simulink model "six_plus_six_AcmsteeringV09_main_2lflm"  (R2014a)
settings: Solver=FixedStepDiscrete  StartTime=0.0  StopTime=10.0  FixedStep=0.0005  RelTol=1e-3
InitFcn:
  | Veh_Par_wxt
undefined symbols (not defined in the file or in its folder): acc_spdctl, ag_thr, B, bra_em, bra_pre_gz2, bra_pre_gz34, bra_pre_yd, brakepre_dem_data, brakeTrq_dem_data, bratrq_max, ecucoder_acal, eff_tran, ESP_switch, G, guzhang_lf, guzhang_lm, guzhang_lr, guzhang_rf, guzhang_rm, guzhang_rr, kd1, kd2, ki1, ki2, kp1, kp2, L, myFIS, premax, Radius, RC_switch, s_opt_yi, s_opt_zhuan, s_opt_zhuan_add, s_opt_zhuan_table, spd_map_mot, spd_spdctl, speed_thr_park, TCS_switch, tras_ratio, trq_map_mot, trqmax_yd, trqmax_zx, trqmaxneg, v_gain, v_table, v_thr_park, zhidong_bianmazhi, zhidong_down, zhidong_up, zhidong_youmen, zhuanxiang_bianmazhi, zhuanxiang_down, zhuanxiang_up, zhuanxiang_youmen
libraries: simulink x980, ec5744lib x59, fuzblock x2
(part 23 of 25)

== system six_plus_six_AcmsteeringV09_main_2lflm/MainControl/mode_control/backward/backward/Drive/驱动防滑控制TCS/直行TCS/Subsystem6 ==
  speed_act_lf : Inport
  speed_act_lm : Inport  Port=2
  speed_act_lr : Inport  Port=3
  Gain : Gain  Gain=1/tras_ratio
  Gain1 : Gain  Gain=pi/30
  Gain2 : Gain  Gain=Radius
  Gain3 : Gain  Gain=3.6
  Gain4 : Gain  Gain=v_gain
  MinMax : MinMax  Inputs=3
  v_act_l : Outport
  wires:
  speed_act_lm/1 -> MinMax/2
  speed_act_lr/1 -> MinMax/3
  speed_act_lf/1 -> MinMax/1
  MinMax/1 -> Gain/1
  Gain/1 -> Gain1/1
  Gain1/1 -> Gain2/1
  Gain2/1 -> Gain3/1
  Gain3/1 -> Gain4/1
  Gain4/1 -> v_act_l/1

== system six_plus_six_AcmsteeringV09_main_2lflm/MainControl/mode_control/backward/backward/Drive/驱动防滑控制TCS/直行TCS/Subsystem7 ==
  speed_act_rf : Inport
  speed_act_rm : Inport  Port=2
  speed_act_rr : Inport  Port=3
  Gain : Gain  Gain=1/tras_ratio
  Gain1 : Gain  Gain=pi/30
  Gain2 : Gain  Gain=Radius
  Gain3 : Gain  Gain=3.6
  Gain4 : Gain  Gain=v_gain
  MinMax : MinMax  Inputs=3
  v_act_r : Outport
  wires:
  Gain4/1 -> v_act_r/1
  Gain3/1 -> Gain4/1
  Gain2/1 -> Gain3/1
  Gain1/1 -> Gain2/1
  Gain/1 -> Gain1/1
  MinMax/1 -> Gain/1
  speed_act_rf/1 -> MinMax/1
  speed_act_rr/1 -> MinMax/3
  speed_act_rm/1 -> MinMax/2

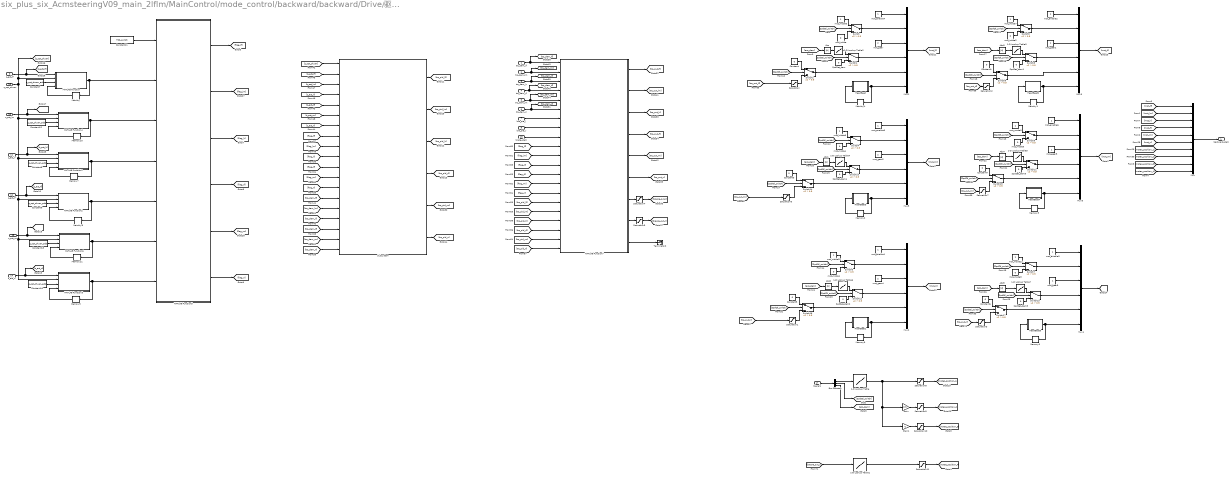
== system six_plus_six_AcmsteeringV09_main_2lflm/MainControl/mode_control/backward/backward/Drive/驱动防滑控制TCS/直行TCS/直行 ==
  trq_dem_lf : Inport
  trq_dem_lm : Inport  Port=2
  trq_dem_lr : Inport  Port=3
  trq_dem_rf : Inport  Port=4
  trq_dem_rm : Inport  Port=5
  trq_dem_rr : Inport  Port=6
  bra_pre_l : Inport  Port=7
  bra_pre_r : Inport  Port=8
  s_act_lf : Inport  Port=9
  s_act_lm : Inport  Port=10
  s_act_lr : Inport  Port=11
  s_act_rf : Inport  Port=12
  s_act_rm : Inport  Port=13
  s_act_rr : Inport  Port=14
  brake_dem : Inport  Port=15
  s_opt_zhuan : Inport  Port=16
  Signals : Inport  Port=17
  1-D Lookup Table : Lookup_n-D  NumberOfTableDimensions=1  BreakpointsForDimension1=zhuanxiang_youmen  Table=zhuanxiang_bianmazhi  InternalRulePriority=Speed  RndMeth=Simplest  InputSameDT=on
  1-D Lookup Table1 : Lookup_n-D  NumberOfTableDimensions=1  BreakpointsForDimension1=zhidong_youmen  Table=zhidong_bianmazhi  InternalRulePriority=Speed  RndMeth=Simplest  InputSameDT=on
  1-D Lookup Table{2..7} (6 alike) : Lookup_n-D  NumberOfTableDimensions=1  BreakpointsForDimension1=acc_spdctl  Table=spd_spdctl  InternalRulePriority=Speed  RndMeth=Simplest  InputSameDT=on
  Abs{,1..5} (6 alike) : Abs
  Bus Selector : BusSelector  OutputSignals=RemoteControl_dem.steer_dem,RemoteControl_dem.SpdCtl_switch,RemoteControl_dem.acc_dem
  Constant{,1,3..6} (6 alike) : Constant  Value=0  OutDataTypeStr=single  SampleTime=-1
  Constant{7..10,12..13} (6 alike) : Constant  Value=s_opt_zhuan_add  OutDataTypeStr=single  SampleTime=-1
  Constant11 : Constant  Value=TCS_switch  OutDataTypeStr=single  SampleTime=-1
  Gain : Gain  Gain=0.5
  Gain1 : Gain  Gain=-1
  HeartBeat : MATLAB Function  TreatAsAtomicUnit=on
  HeartBeat1 : MATLAB Function  TreatAsAtomicUnit=on
  HeartBeat2 : MATLAB Function  TreatAsAtomicUnit=on
  HeartBeat3 : MATLAB Function  TreatAsAtomicUnit=on
  HeartBeat4 : MATLAB Function  TreatAsAtomicUnit=on
  HeartBeat5 : MATLAB Function  TreatAsAtomicUnit=on
  MATLAB Function : MATLAB Function  TreatAsAtomicUnit=on
  MATLAB Function1 : MATLAB Function  TreatAsAtomicUnit=on
  MATLAB Function2 : MATLAB Function  TreatAsAtomicUnit=on
  MATLAB Function3 : MATLAB Function  TreatAsAtomicUnit=on
  MATLAB Function4 : MATLAB Function  TreatAsAtomicUnit=on
  MATLAB Function5 : MATLAB Function  TreatAsAtomicUnit=on
  MATLAB Function6 : MATLAB Function  TreatAsAtomicUnit=on
  MATLAB Function7 : MATLAB Function  TreatAsAtomicUnit=on
  Memory{,1..11} (12 alike) : Memory  InheritSampleTime=on
  Mux : Mux  Inputs=10
  Mux{1..6} (6 alike) : Mux  Inputs=6
  Saturation{,1..3,6..7} (6 alike) : Saturate  UpperLimit=trqmax_zx  LowerLimit=trqmaxneg  OutDataTypeStr=single
  Saturation10 : Saturate  UpperLimit=zhuanxiang_up  LowerLimit=zhuanxiang_down
  Saturation11 : Saturate  UpperLimit=zhidong_up  LowerLimit=zhidong_down
  Saturation4 : Saturate  UpperLimit=premax  LowerLimit=0
  Saturation5 : Saturate  UpperLimit=premax  LowerLimit=0
  Saturation8 : Saturate  UpperLimit=zhuanxiang_up  LowerLimit=zhuanxiang_down
  Saturation9 : Saturate  UpperLimit=zhuanxiang_up  LowerLimit=zhuanxiang_down
  SpdSet_dem{,1..5} (6 alike) : Constant  Value=0  OutDataTypeStr=single  SampleTime=-1
  Subsystem : Subsystem
  Switch{,1..17} (18 alike) : Switch  Criteria=u2 > Threshold  Threshold=0.5
  Terminator2 : Terminator
  mot_enable{1..6} (6 alike) : Constant  OutDataTypeStr=single  SampleTime=-1
  mot_gear : Constant  Value=2  OutDataTypeStr=single  SampleTime=-1
  mot_gear1 : Constant  OutDataTypeStr=single  SampleTime=-1
  mot_gear2 : Constant  Value=2  OutDataTypeStr=single  SampleTime=-1
  mot_gear3 : Constant  OutDataTypeStr=single  SampleTime=-1
  mot_gear4 : Constant  Value=2  OutDataTypeStr=single  SampleTime=-1
  mot_gear5 : Constant  OutDataTypeStr=single  SampleTime=-1
  mot_mode{,1..5} (6 alike) : Constant  Value=0  OutDataTypeStr=single  SampleTime=-1
  mot_mode{6..11} (6 alike) : Constant  OutDataTypeStr=single  SampleTime=-1
  backward_dem : Outport
  wires:
  Mux/1 -> backward_dem/1
  Memory4/1 -> HeartBeat/1(life_pre)
  HeartBeat/1(life) -> Memory4/1, Mux1/6
  Mux1/1 -> [mot_lf]
  [trq_out_lf] -> Saturation/1
  mot_gear/1 -> Mux1/3
  mot_enable4/1 -> Mux1/1
  Switch1/1 -> Mux1/4
  Memory1/1 -> HeartBeat2/1(life_pre)
  HeartBeat2/1(life) -> Mux3/6, Memory1/1
  Mux3/1 -> [mot_rf]
  [trq_out_rf] -> Saturation2/1
  Switch3/1 -> Mux3/2
  mot_gear1/1 -> Mux3/3
  mot_enable2/1 -> Mux3/1
  Switch8/1 -> Mux3/4
  Memory2/1 -> HeartBeat3/1(life_pre)
  HeartBeat3/1(life) -> Mux5/6, Memory2/1
  Mux5/1 -> [mot_lm]
  [trq_out_lm] -> Saturation6/1
  Switch4/1 -> Mux5/2
  mot_gear2/1 -> Mux5/3
  mot_enable5/1 -> Mux5/1
  Switch10/1 -> Mux5/4
  Memory3/1 -> HeartBeat4/1(life_pre)
  HeartBeat4/1(life) -> Memory3/1, Mux6/6
  Mux6/1 -> [mot_rm]
  [trq_out_rm] -> Saturation7/1
  Switch5/1 -> Mux6/2
  mot_gear3/1 -> Mux6/3
  mot_enable6/1 -> Mux6/1
  Switch11/1 -> Mux6/4
  Memory5/1 -> HeartBeat1/1(life_pre)
  HeartBeat1/1(life) -> Mux2/6, Memory5/1
  Mux2/1 -> [mot_lr]
  [trq_out_lr] -> Saturation1/1
  Switch6/1 -> Mux2/2
  mot_gear4/1 -> Mux2/3
  mot_enable1/1 -> Mux2/1
  Switch12/1 -> Mux2/4
  Memory6/1 -> HeartBeat5/1(life_pre)
  HeartBeat5/1(life) -> Memory6/1, Mux4/6
  Mux4/1 -> [mot_rr]
  [trq_out_rr] -> Saturation3/1
  Switch7/1 -> Mux4/2
  mot_gear5/1 -> Mux4/3
  mot_enable3/1 -> Mux4/1
  Switch13/1 -> Mux4/4
  [mot_lf] -> Mux/1
  [mot_lm] -> Mux/2
  [mot_lr] -> Mux/3
  [mot_rf] -> Mux/4
  [mot_rm] -> Mux/5
  [mot_rr] -> Mux/6
  [motec_position_1] -> Mux/7
  [motec_position_2] -> Mux/8
  [motec_position_3] -> Mux/9
  1-D Lookup Table1/1 -> Saturation11/1
  1-D Lookup Table/1 -> Gain1/1, Gain/1, Saturation8/1
  Signals/1 -> Bus Selector/1
  Gain1/1 -> Saturation10/1
  Bus Selector/1 -> 1-D Lookup Table/1  "<steer_dem>"
  Gain/1 -> Saturation9/1
  Saturation8/1 -> [motec_position_1]
  Saturation9/1 -> [motec_position_2]
  Saturation10/1 -> [motec_position_3]
  Saturation11/1 -> [motec_position_4]
  [brapre_out_l] -> 1-D Lookup Table1/1
  [motec_position_4] -> Mux/10
  Bus Selector/2 -> [SpdCtl_switch]  "<SpdCtl_switch>"
  [SpdCtl_switch] -> Switch/2
  mot_mode6/1 -> Switch/1
  mot_mode/1 -> Switch/3
  Switch/1 -> Mux1/2
  [SpdCtl_switch] -> Switch1/2
  SpdSet_dem/1 -> Switch1/3
  Bus Selector/3 -> [acc_dem]  "<acc_dem>"
  [acc_dem] -> Abs/1
  1-D Lookup Table2/1 -> Switch1/1
  [SpdCtl_switch] -> Switch2/2
  Saturation/1 -> Switch2/3
  Constant/1 -> Switch2/1
  Switch2/1 -> Mux1/5
  [SpdCtl_switch] -> Switch3/2
  mot_mode7/1 -> Switch3/1
  mot_mode2/1 -> Switch3/3
  [SpdCtl_switch] -> Switch4/2
  mot_mode8/1 -> Switch4/1
  mot_mode4/1 -> Switch4/3
  [SpdCtl_switch] -> Switch5/2
  mot_mode9/1 -> Switch5/1
  mot_mode5/1 -> Switch5/3
  [SpdCtl_switch] -> Switch6/2
  mot_mode10/1 -> Switch6/1
  mot_mode1/1 -> Switch6/3
  [SpdCtl_switch] -> Switch7/2
  mot_mode11/1 -> Switch7/1
  mot_mode3/1 -> Switch7/3
  [SpdCtl_switch] -> Switch8/2
  [acc_dem] -> Abs3/1
  1-D Lookup Table3/1 -> Switch8/1
  SpdSet_dem1/1 -> Switch8/3
  [SpdCtl_switch] -> Switch9/2
  Constant1/1 -> Switch9/1
  Saturation2/1 -> Switch9/3
  Switch9/1 -> Mux3/5
  [SpdCtl_switch] -> Switch10/2
  [acc_dem] -> Abs1/1
  1-D Lookup Table4/1 -> Switch10/1
  SpdSet_dem4/1 -> Switch10/3
  [SpdCtl_switch] -> Switch11/2
  [acc_dem] -> Abs4/1
  1-D Lookup Table5/1 -> Switch11/1
  SpdSet_dem5/1 -> Switch11/3
  [SpdCtl_switch] -> Switch12/2
  [acc_dem] -> Abs2/1
  1-D Lookup Table6/1 -> Switch12/1
  SpdSet_dem2/1 -> Switch12/3
  [SpdCtl_switch] -> Switch13/2
  [acc_dem] -> Abs5/1
  1-D Lookup Table7/1 -> Switch13/1
  SpdSet_dem3/1 -> Switch13/3
  [SpdCtl_switch] -> Switch14/2
  Constant3/1 -> Switch14/1
  Saturation6/1 -> Switch14/3
  Switch14/1 -> Mux5/5
  [SpdCtl_switch] -> Switch15/2
  Constant4/1 -> Switch15/1
  Saturation7/1 -> Switch15/3
  Switch15/1 -> Mux6/5
  [SpdCtl_switch] -> Switch16/2
  Constant5/1 -> Switch16/1
  Saturation1/1 -> Switch16/3
  Switch16/1 -> Mux2/5
  [SpdCtl_switch] -> Switch17/2
  Constant6/1 -> Switch17/1
  Saturation3/1 -> Switch17/3
  Switch17/1 -> Mux4/5
  Constant10/1 -> MATLAB Function3/3(s_opt_zhuan_add)
  Memory9/1 -> MATLAB Function3/4(flag_rr_pre)
  MATLAB Function3/1(flag_rr) -> Memory9/1, MATLAB Function5/7(flag_rr)
  s_act_rr/1 -> [s_act_rr], MATLAB Function3/1(s_act_rr)
  Constant9/1 -> MATLAB Function2/3(s_opt_zhuan_add)
  Memory8/1 -> MATLAB Function2/4(flag_rf_pre)
  MATLAB Function2/1(flag_rf) -> Memory8/1, MATLAB Function5/5(flag_rf)
  s_act_rf/1 -> MATLAB Function2/1(s_act_rf), [s_act_rf]
  Constant8/1 -> MATLAB Function1/3(s_opt_zhuan_add)
  Memory7/1 -> MATLAB Function1/4(flag_lr_pre)
  MATLAB Function1/1(flag_lr) -> Memory7/1, MATLAB Function5/4(flag_lr)
  s_act_lr/1 -> [s_act_lr], MATLAB Function1/1(s_act_lr)
  Constant7/1 -> MATLAB Function/3(s_opt_zhuan_add)
  Memory/1 -> MATLAB Function/4(flag_lf_pre)
  MATLAB Function/1(flag_lf) -> Memory/1, MATLAB Function5/2(flag_lf)
  s_act_lf/1 -> [s_act_lf], MATLAB Function/1(s_act_lf)
  [trq_dem_lf] -> Subsystem/14(trq_dem_lf)
  [flag_lf] -> Subsystem/8(flag_lf)
  [trq_dem_rf] -> Subsystem/17(trq_dem_rf)
  [trq_dem_lr] -> Subsystem/16(trq_dem_lr)
  [flag_lr] -> Subsystem/10(flag_lr)
  [flag_rf] -> Subsystem/11(flag_rf)
  [trq_dem_rr] -> Subsystem/19(trq_dem_rr)
  [flag_rr] -> Subsystem/13(flag_rr)
  [s_opt_zhuan] -> Subsystem/1(s_opt_zhuan)
  [s_act_rr] -> Subsystem/7(s_act_rr)
  [s_act_rf] -> Subsystem/5(s_act_rf)
  [s_act_lr] -> Subsystem/4(s_act_lr)
  [s_act_lf] -> Subsystem/2(s_act_lf)
  Subsystem/3(trq_pid_lr) -> [trq_pid_lr]
  Subsystem/1(trq_pid_lf) -> [trq_pid_lf]
  Subsystem/6(trq_pid_rr) -> [trq_pid_rr]
  Subsystem/4(trq_pid_rf) -> [trq_pid_rf]
  MATLAB Function5/1(flag_lf1) -> [flag_lf]
  MATLAB Function5/3(flag_lr1) -> [flag_lr]
  MATLAB Function5/4(flag_rf1) -> [flag_rf]
  MATLAB Function5/6(flag_rr1) -> [flag_rr]
  Constant12/1 -> MATLAB Function4/3(s_opt_zhuan_add)
  Memory10/1 -> MATLAB Function4/4(flag_lm_pre)
  MATLAB Function4/1(flag_lm) -> MATLAB Function5/3(flag_lm), Memory10/1
  s_act_lm/1 -> MATLAB Function4/1(s_act_lm), [s_act_lm]
  Constant13/1 -> MATLAB Function6/3(s_opt_zhuan_add)
  Memory11/1 -> MATLAB Function6/4(flag_rm_pre)
  MATLAB Function6/1(flag_rm) -> Memory11/1, MATLAB Function5/6(flag_rm)
  s_act_rm/1 -> [s_act_rm], MATLAB Function6/1(s_act_rm)
  s_opt_zhuan/1 -> MATLAB Function/2(s_opt_zhuan), [s_opt_zhuan], MATLAB Function4/2(s_opt_zhuan), MATLAB Function1/2(s_opt_zhuan), MATLAB Function2/2(s_opt_zhuan), MATLAB Function6/2(s_opt_zhuan), MATLAB Function3/2(s_opt_zhuan)
  MATLAB Function5/2(flag_lm1) -> [flag_lm]
  MATLAB Function5/5(flag_rm1) -> [flag_rm]
  Constant11/1 -> MATLAB Function5/1(TCS_switch)
  [s_act_lm] -> Subsystem/3(s_act_lm)
  [s_act_rm] -> Subsystem/6(s_act_rm)
  [flag_lm] -> Subsystem/9(flag_lm)
  [flag_rm] -> Subsystem/12(flag_rm)
  [trq_dem_lm] -> Subsystem/15(trq_dem_lm)
  [trq_dem_rm] -> Subsystem/18(trq_dem_rm)
  Subsystem/2(trq_pid_lm) -> [trq_pid_lm]
  Subsystem/5(trq_pid_rm) -> [trq_pid_rm]
  [flag_rr] -> MATLAB Function7/15(flag_rr)
  [flag_rf] -> MATLAB Function7/13(flag_rf)
  [flag_lr] -> MATLAB Function7/12(flag_lr)
  [flag_lf] -> MATLAB Function7/10(flag_lf)
  [trq_pid_lf] -> MATLAB Function7/16(trq_pid_lf)
  [trq_pid_lr] -> MATLAB Function7/18(trq_pid_lr)
  [trq_pid_rf] -> MATLAB Function7/19(trq_pid_rf)
  [trq_pid_rr] -> MATLAB Function7/21(trq_pid_rr)
  trq_dem_lf/1 -> MATLAB Function7/1(trq_dem_lf), [trq_dem_lf]
  trq_dem_lr/1 -> [trq_dem_lr], MATLAB Function7/3(trq_dem_lr)
  trq_dem_rf/1 -> MATLAB Function7/4(trq_dem_rf), [trq_dem_rf]
  trq_dem_rr/1 -> [trq_dem_rr], MATLAB Function7/6(trq_dem_rr)
  bra_pre_l/1 -> MATLAB Function7/7(bra_pre_l)
  bra_pre_r/1 -> MATLAB Function7/8(bra_pre_r)
  MATLAB Function7/1(trq_out_lf) -> [trq_out_lf]
  MATLAB Function7/3(trq_out_lr) -> [trq_out_lr]
  MATLAB Function7/4(trq_out_rf) -> [trq_out_rf]
  MATLAB Function7/6(trq_out_rr) -> [trq_out_rr]
  MATLAB Function7/7(brapre_out_l) -> Saturation4/1
  MATLAB Function7/8(brapre_out_r) -> Saturation5/1
  brake_dem/1 -> MATLAB Function7/9(brake_dem)
  MATLAB Function7/9(mode) -> Terminator2/1
  Saturation4/1 -> [brapre_out_l]
  Saturation5/1 -> [brapre_out_r]
  MATLAB Function7/2(trq_out_lm) -> [trq_out_lm]
  MATLAB Function7/5(trq_out_rm) -> [trq_out_rm]
  trq_dem_lm/1 -> [trq_dem_lm], MATLAB Function7/2(trq_dem_lm)
  trq_dem_rm/1 -> [trq_dem_rm], MATLAB Function7/5(trq_dem_rm)
  [flag_lm] -> MATLAB Function7/11(flag_lm)
  [flag_rm] -> MATLAB Function7/14(flag_rm)
  [trq_pid_lm] -> MATLAB Function7/17(trq_pid_lm)
  [trq_pid_rm] -> MATLAB Function7/20(trq_pid_rm)
  Abs/1 -> 1-D Lookup Table2/1
  Abs1/1 -> 1-D Lookup Table4/1
  Abs2/1 -> 1-D Lookup Table6/1
  Abs3/1 -> 1-D Lookup Table3/1
  Abs4/1 -> 1-D Lookup Table5/1
  Abs5/1 -> 1-D Lookup Table7/1

== system six_plus_six_AcmsteeringV09_main_2lflm/MainControl/mode_control/forward/forward/Drive/驱动防滑控制TCS/直行TCS/Subsystem ==
  speed_act_lf : Inport
  v_act : Inport  Port=2
  Add : Sum
  Constant : Constant  Value=eps  OutDataTypeStr=single  SampleTime=-1
  Divide : Product  Inputs=*/
  Gain : Gain  Gain=pi/30
  Gain1 : Gain  Gain=Radius
  Gain2 : Gain  Gain=1/3.6
  Gain3 : Gain  Gain=1/tras_ratio
  Subtract : Sum  Inputs=+-
  s_act_lf : Outport
  wires:
  Divide/1 -> s_act_lf/1
  Add/1 -> Divide/2
  Constant/1 -> Add/2
  Subtract/1 -> Divide/1
  Gain1/1 -> Subtract/1, Add/1
  v_act/1 -> Gain2/1
  Gain/1 -> Gain1/1
  speed_act_lf/1 -> Gain3/1
  Gain3/1 -> Gain/1
  Gain2/1 -> Subtract/2

== system six_plus_six_AcmsteeringV09_main_2lflm/MainControl/mode_control/forward/forward/Drive/驱动防滑控制TCS/直行TCS/Subsystem1 ==
  speed_act_lm : Inport
  v_act : Inport  Port=2
  Add : Sum
  Constant : Constant  Value=eps  OutDataTypeStr=single  SampleTime=-1
  Divide : Product  Inputs=*/
  Gain : Gain  Gain=pi/30
  Gain1 : Gain  Gain=Radius
  Gain2 : Gain  Gain=1/3.6
  Gain3 : Gain  Gain=1/tras_ratio
  Subtract : Sum  Inputs=+-
  s_act_lm : Outport
  wires:
  Gain2/1 -> Subtract/2
  Gain3/1 -> Gain/1
  speed_act_lm/1 -> Gain3/1
  Gain/1 -> Gain1/1
  v_act/1 -> Gain2/1
  Gain1/1 -> Add/1, Subtract/1
  Subtract/1 -> Divide/1
  Constant/1 -> Add/2
  Add/1 -> Divide/2
  Divide/1 -> s_act_lm/1

== system six_plus_six_AcmsteeringV09_main_2lflm/MainControl/mode_control/forward/forward/Drive/驱动防滑控制TCS/直行TCS/Subsystem2 ==
  speed_act_lr : Inport
  v_act : Inport  Port=2
  Add : Sum
  Constant : Constant  Value=eps  OutDataTypeStr=single  SampleTime=-1
  Divide : Product  Inputs=*/
  Gain : Gain  Gain=pi/30
  Gain1 : Gain  Gain=Radius
  Gain2 : Gain  Gain=1/3.6
  Gain3 : Gain  Gain=1/tras_ratio
  Subtract : Sum  Inputs=+-
  s_act_lr : Outport
  wires:
  Gain2/1 -> Subtract/2
  Gain3/1 -> Gain/1
  speed_act_lr/1 -> Gain3/1
  Gain/1 -> Gain1/1
  v_act/1 -> Gain2/1
  Gain1/1 -> Add/1, Subtract/1
  Subtract/1 -> Divide/1
  Constant/1 -> Add/2
  Add/1 -> Divide/2
  Divide/1 -> s_act_lr/1

== system six_plus_six_AcmsteeringV09_main_2lflm/MainControl/mode_control/forward/forward/Drive/驱动防滑控制TCS/直行TCS/Subsystem3 ==
  speed_act_rf : Inport
  v_act : Inport  Port=2
  Add : Sum
  Constant : Constant  Value=eps  OutDataTypeStr=single  SampleTime=-1
  Divide : Product  Inputs=*/
  Gain : Gain  Gain=pi/30
  Gain1 : Gain  Gain=Radius
  Gain2 : Gain  Gain=1/3.6
  Gain3 : Gain  Gain=1/tras_ratio
  Subtract : Sum  Inputs=+-
  s_act_rf : Outport
  wires:
  Divide/1 -> s_act_rf/1
  Add/1 -> Divide/2
  Constant/1 -> Add/2
  Subtract/1 -> Divide/1
  Gain1/1 -> Subtract/1, Add/1
  v_act/1 -> Gain2/1
  Gain/1 -> Gain1/1
  speed_act_rf/1 -> Gain3/1
  Gain3/1 -> Gain/1
  Gain2/1 -> Subtract/2

== system six_plus_six_AcmsteeringV09_main_2lflm/MainControl/mode_control/forward/forward/Drive/驱动防滑控制TCS/直行TCS/Subsystem4 ==
  speed_act_rm : Inport
  v_act : Inport  Port=2
  Add : Sum
  Constant : Constant  Value=eps  OutDataTypeStr=single  SampleTime=-1
  Divide : Product  Inputs=*/
  Gain : Gain  Gain=pi/30
  Gain1 : Gain  Gain=Radius
  Gain2 : Gain  Gain=1/3.6
  Gain3 : Gain  Gain=1/tras_ratio
  Subtract : Sum  Inputs=+-
  s_act_rm : Outport
  wires:
  Gain2/1 -> Subtract/2
  Gain3/1 -> Gain/1
  speed_act_rm/1 -> Gain3/1
  Gain/1 -> Gain1/1
  v_act/1 -> Gain2/1
  Gain1/1 -> Add/1, Subtract/1
  Subtract/1 -> Divide/1
  Constant/1 -> Add/2
  Add/1 -> Divide/2
  Divide/1 -> s_act_rm/1

== system six_plus_six_AcmsteeringV09_main_2lflm/MainControl/mode_control/forward/forward/Drive/驱动防滑控制TCS/直行TCS/Subsystem5 ==
  speed_act_rr : Inport
  v_act : Inport  Port=2
  Add : Sum
  Constant : Constant  Value=eps  OutDataTypeStr=single  SampleTime=-1
  Divide : Product  Inputs=*/
  Gain : Gain  Gain=pi/30
  Gain1 : Gain  Gain=Radius
  Gain2 : Gain  Gain=1/3.6
  Gain3 : Gain  Gain=1/tras_ratio
  Subtract : Sum  Inputs=+-
  s_act_rr : Outport
  wires:
  Divide/1 -> s_act_rr/1
  Add/1 -> Divide/2
  Constant/1 -> Add/2
  Subtract/1 -> Divide/1
  Gain1/1 -> Subtract/1, Add/1
  v_act/1 -> Gain2/1
  Gain/1 -> Gain1/1
  speed_act_rr/1 -> Gain3/1
  Gain3/1 -> Gain/1
  Gain2/1 -> Subtract/2

== system six_plus_six_AcmsteeringV09_main_2lflm/MainControl/mode_control/forward/forward/Drive/驱动防滑控制TCS/直行TCS/Subsystem6 ==
  speed_act_lf : Inport
  speed_act_lm : Inport  Port=2
  speed_act_lr : Inport  Port=3
  Gain : Gain  Gain=1/tras_ratio
  Gain1 : Gain  Gain=pi/30
  Gain2 : Gain  Gain=Radius
  Gain3 : Gain  Gain=3.6
  Gain4 : Gain  Gain=v_gain
  MinMax : MinMax  Inputs=3
  v_act_l : Outport
  wires:
  speed_act_lm/1 -> MinMax/2
  speed_act_lr/1 -> MinMax/3
  speed_act_lf/1 -> MinMax/1
  MinMax/1 -> Gain/1
  Gain/1 -> Gain1/1
  Gain1/1 -> Gain2/1
  Gain2/1 -> Gain3/1
  Gain3/1 -> Gain4/1
  Gain4/1 -> v_act_l/1

== system six_plus_six_AcmsteeringV09_main_2lflm/MainControl/mode_control/forward/forward/Drive/驱动防滑控制TCS/直行TCS/Subsystem7 ==
  speed_act_rf : Inport
  speed_act_rm : Inport  Port=2
  speed_act_rr : Inport  Port=3
  Gain : Gain  Gain=1/tras_ratio
  Gain1 : Gain  Gain=pi/30
  Gain2 : Gain  Gain=Radius
  Gain3 : Gain  Gain=3.6
  Gain4 : Gain  Gain=v_gain
  MinMax : MinMax  Inputs=3
  v_act_r : Outport
  wires:
  Gain4/1 -> v_act_r/1
  Gain3/1 -> Gain4/1
  Gain2/1 -> Gain3/1
  Gain1/1 -> Gain2/1
  Gain/1 -> Gain1/1
  MinMax/1 -> Gain/1
  speed_act_rf/1 -> MinMax/1
  speed_act_rr/1 -> MinMax/3
  speed_act_rm/1 -> MinMax/2

== matlab function six_plus_six_AcmsteeringV09_main_2lflm/MainControl/mode_control/neutral/neutral/HeartBeat ==
  data: life_pre input; life output
function life = fcn(life_pre)
%#codegen
life=single(life_pre+1);
if life>255
    life=single(0);
end
end

== matlab function six_plus_six_AcmsteeringV09_main_2lflm/MainControl/mode_control/neutral/neutral/HeartBeat1 ==
  data: life_pre input; life output
function life = fcn(life_pre)
%#codegen
life=single(life_pre+1);
if life>255
    life=single(0);
end
end

== matlab function six_plus_six_AcmsteeringV09_main_2lflm/MainControl/mode_control/neutral/neutral/HeartBeat2 ==
  data: life_pre input; life output
function life = fcn(life_pre)
%#codegen
life=single(life_pre+1);
if life>255
    life=single(0);
end
end

== matlab function six_plus_six_AcmsteeringV09_main_2lflm/MainControl/mode_control/backward/backward/Brake/HeartBeat ==
  data: life_pre input; life output
function life = fcn(life_pre)
%#codegen
life=single(life_pre+1);
if life>255
    life=single(0);
end
end

== matlab function six_plus_six_AcmsteeringV09_main_2lflm/MainControl/mode_control/backward/backward/Brake/HeartBeat2 ==
  data: life_pre input; life output
function life = fcn(life_pre)
%#codegen
life=single(life_pre+1);
if life>255
    life=single(0);
end
end

== matlab function six_plus_six_AcmsteeringV09_main_2lflm/MainControl/mode_control/backward/backward/Brake/HeartBeat4 ==
  data: life_pre input; life output
function life = fcn(life_pre)
%#codegen
life=single(life_pre+1);
if life>255
    life=single(0);
end
end

== matlab function six_plus_six_AcmsteeringV09_main_2lflm/MainControl/mode_control/backward/backward/Brake/Switch Case Action Subsystem/MATLAB Function5 ==
  data: bratrq_dem_lf input; bratrq_dem_lm input; bratrq_dem_lr input; bratrq_dem_rf input; bratrq_dem_rm input; bratrq_dem_rr input; pwr_chg_bat input; bratrq_mot_lf output; bratrq_mot_lm output; pwr_chg_bat1 input; pwr_chg_bat2 input; trqlimL_dig_lf input; bratrq_mot_lr output; bratrq_mot_rf output; bratrq_mot_rm output; bratrq_mot_rr output; trqlimL_dig_lm input; trqlimL_dig_lr input; trqlimL_dig_rf input; trqlimL_dig_rm input; trqlimL_dig_rr input; speed_act_lf input; speed_act_lm input; speed_act_lr input; speed_act_rf input; speed_act_rm input; speed_act_rr input; trqlim_map_lf input; brapre_out_l output; brapre_out_r output; trqlim_map_lm input; trqlim_map_lr input; trqlim_map_rf input; trqlim_map_rm input; trqlim_map_rr input; tras_ratio input; guzhang_lf input; guzhang_lm input; guzhang_lr input; guzhang_rf input; guzhang_rm input; guzhang_rr input
function [bratrq_mot_lf,bratrq_mot_lm,bratrq_mot_lr,bratrq_mot_rf,bratrq_mot_rm,bratrq_mot_rr,brapre_out_l,brapre_out_r] = fcn(bratrq_dem_lf,bratrq_dem_lm,bratrq_dem_lr,bratrq_dem_rf,bratrq_dem_rm,bratrq_dem_rr,pwr_chg_bat,pwr_chg_bat1,pwr_chg_bat2,trqlimL_dig_lf,trqlimL_dig_lm,trqlimL_dig_lr,trqlimL_dig_rf,trqlimL_dig_rm,trqlimL_dig_rr,speed_act_lf,speed_act_lm,speed_act_lr,speed_act_rf,speed_act_rm,speed_act_rr,trqlim_map_lf,trqlim_map_lm,trqlim_map_lr,trqlim_map_rf,trqlim_map_rm,trqlim_map_rr,tras_ratio,guzhang_lf,guzhang_lm,guzhang_lr,guzhang_rf,guzhang_rm,guzhang_rr)
%#codegen pid模块在外面做，里面进行十六种情况的判断，先看一下效果，不能再修改。前轴单独控制，后轴低选控制

bratrq_mot_lf1=single(bratrq_dem_lf/tras_ratio);
bratrq_mot_lf2=single(9549*(pwr_chg_bat/2)/speed_act_lf);
bratrq_mot_lf=single(min(trqlimL_dig_lf,min(bratrq_mot_lf1,bratrq_mot_lf2)));

bratrq_mot_lm1=single(bratrq_dem_lm/tras_ratio);
bratrq_mot_lm2=single(9549*(pwr_chg_bat1/2)/speed_act_lm);
bratrq_mot_lm=single(min(trqlimL_dig_lm,min(bratrq_mot_lm1,bratrq_mot_lm2)));

bratrq_mot_lr1=single(bratrq_dem_lr/tras_ratio);
bratrq_mot_lr2=single(9549*(pwr_chg_bat2/2)/speed_act_lr);
bratrq_mot_lr=single(min(trqlimL_dig_lr,min(bratrq_mot_lr1,bratrq_mot_lr2)));
 
bratrq_mot_rf1=single(bratrq_dem_rf/tras_ratio);
bratrq_mot_rf2=single(9549*(pwr_chg_bat/2)/speed_act_rf);
bratrq_mot_rf=single(min(trqlimL_dig_rf,min(bratrq_mot_rf1,bratrq_mot_rf2)));

bratrq_mot_rm1=single(bratrq_dem_rm/tras_ratio);
bratrq_mot_rm2=single(9549*(pwr_chg_bat1/2)/speed_act_rm);
bratrq_mot_rm=single(min(trqlimL_dig_rm,min(bratrq_mot_rm1,bratrq_mot_rm2)));

bratrq_mot_rr1=single(bratrq_dem_rr/tras_ratio);
bratrq_mot_rr2=single(9549*(pwr_chg_bat2/2)/speed_act_rr);
bratrq_mot_rr=single(min(trqlimL_dig_rr,min(bratrq_mot_rr1,bratrq_mot_rr2)));

brapre_out_l=single(((bratrq_dem_lf+bratrq_dem_lm+bratrq_dem_lr)-(bratrq_mot_lf+bratrq_mot_lm+bratrq_mot_lr)*tras_ratio)/3/150);
brapre_out_r=single(((bratrq_dem_rf+bratrq_dem_rm+bratrq_dem_rr)-(bratrq_mot_rf+bratrq_mot_rm+bratrq_mot_rr)*tras_ratio)/3/150);







bratrq_mot_lf=single(min(bratrq_mot_lf,trqlim_map_lf));%限一下最大值在外特性内，最小值大于0
bratrq_mot_lf=single(max(bratrq_mot_lf,0));
bratrq_mot_lr=single(min(bratrq_mot_lr,trqlim_map_lr));
bratrq_mot_lr=single(max(bratrq_mot_lr,0));
bratrq_mot_rf=single(min(bratrq_mot_rf,trqlim_map_rf));
bratrq_mot_rf=single(max(bratrq_mot_rf,0));
bratrq_mot_rr=single(min(bratrq_mot_rr,trqlim_map_rr));
bratrq_mot_rr=single(max(bratrq_mot_rr,0));

% brapre_out_l=brapre_out_l;
% brapre_out_r=brapre_out_r;
brapre_out_l=single(brapre_out_l*150/125);%第二辆车的制动压力与制动力的关系调整一下。
brapre_out_r=single(brapre_out_r*150/125);

if guzhang_lf==1
    bratrq_mot_lf=single(0);
end
if guzhang_lm==1
    bratrq_mot_lm=single(0);
end
if guzhang_lr==1
    bratrq_mot_lr=single(0);
end
if guzhang_rf==1
    bratrq_mot_rf=single(0);
end
if guzhang_rm==1
    bratrq_mot_rm=single(0);
end
if guzhang_rr==1
    bratrq_mot_rr=single(0);
end

end

== matlab function six_plus_six_AcmsteeringV09_main_2lflm/MainControl/mode_control/center_steer/center_steer/HeartBeat4 ==
  data: life_pre input; life output
function life = fcn(life_pre)
%#codegen
life=single(life_pre+1);
if life>255
    life=single(0);
end
end

== matlab function six_plus_six_AcmsteeringV09_main_2lflm/MainControl/mode_control/emergency_stop/emergency_stop/HeartBeat2 ==
  data: life_pre input; life output
function life = fcn(life_pre)
%#codegen
life=single(life_pre+1);
if life>255
    life=single(0);
end
end

== matlab function six_plus_six_AcmsteeringV09_main_2lflm/MainControl/mode_control/forward/forward/Drive/驱动防滑控制TCS/直行TCS/直行/HeartBeat ==
  data: life_pre input; life output
function life = fcn(life_pre)
%#codegen
life=single(life_pre+1);
if life>255
    life=single(0);
end
end

== matlab function six_plus_six_AcmsteeringV09_main_2lflm/MainControl/mode_switch/mode_switch ==
  data: brake_emerg input; park input; mode_dem_out output int8; acc_dem input; steer_dem input; brake_dem input; center input; MCU0_SpeedFdk input; MCU0_1SpeedFdk input; MCU0_2SpeedFdk input; MCU0_3SpeedFdk input; MCU0_4SpeedFdk input; MCU0_5SpeedFdk input; speed_thr_park input; mode_dem_out_pre input
 function mode_dem_out = fcn(brake_emerg,park,acc_dem,steer_dem,brake_dem,center,MCU0_SpeedFdk,MCU0_1SpeedFdk,MCU0_2SpeedFdk,MCU0_3SpeedFdk,MCU0_4SpeedFdk,MCU0_5SpeedFdk,speed_thr_park,mode_dem_out_pre)
%#codegen
mode_dem_out=int8(mode_dem_out_pre);

if park==1  && MCU0_SpeedFdk<=speed_thr_park && MCU0_1SpeedFdk<=speed_thr_park && MCU0_2SpeedFdk<=speed_thr_park && MCU0_3SpeedFdk<=speed_thr_park  && MCU0_4SpeedFdk<=speed_thr_park  && MCU0_5SpeedFdk<=speed_thr_park && brake_emerg==0
    mode_dem_out=int8(0);
elseif acc_dem>0 && MCU0_SpeedFdk>=0 && MCU0_1SpeedFdk>=0 && MCU0_2SpeedFdk>=0 && MCU0_3SpeedFdk>=0  && MCU0_4SpeedFdk>=0  && MCU0_5SpeedFdk>=0 && brake_emerg==0  && park==0  && center==0
    mode_dem_out=int8(1);
elseif acc_dem==0 && brake_emerg==0  && park==0  && center==0
    mode_dem_out=int8(2);
elseif acc_dem<0 && MCU0_SpeedFdk>=0 && MCU0_1SpeedFdk>=0 && MCU0_2SpeedFdk>=0 && MCU0_3SpeedFdk>=0  && MCU0_4SpeedFdk>=0  && MCU0_5SpeedFdk>=0 && brake_emerg==0  && park==0  && center==0
    mode_dem_out=int8(3);
elseif center==1  && brake_emerg==0  && park==0        
    mode_dem_out=int8(1);
elseif brake_emerg==1
    mode_dem_out=int8(5);   
% else
%     mode_dem_out=int8(5);
end



end

== matlab function six_plus_six_AcmsteeringV09_main_2lflm/Data_input/6/Enabled
Subsystem/MATLAB Function ==
  data: data1 input; y output; data2 input; data3 input; data4 input
function y = fcn(data1,data2,data3,data4)
%#codegen
y1=data4*256^3+data3*256^2+data2*256+data1;
y=typecast(uint32(y1),'single');
end
% y = u;

== matlab function six_plus_six_AcmsteeringV09_main_2lflm/Data_input/9/Enabled Subsystem/MATLAB Function1 ==
  data: data1 input; y output; data2 input; data3 input; data4 input
function y = fcn(data1,data2,data3,data4)
%#codegen
y1=data4*256^3+data3*256^2+data2*256+data1;
% y=typecast(uint32(y1),'single');
y=single(y1*10^-7);
end
% y = u;

== matlab function six_plus_six_AcmsteeringV09_main_2lflm/MainControl/mode_control/Park/park/HeartBeat2 ==
  data: life_pre input; life output
function life = fcn(life_pre)
%#codegen
life=single(life_pre+1);
if life>255
    life=single(0);
end
end

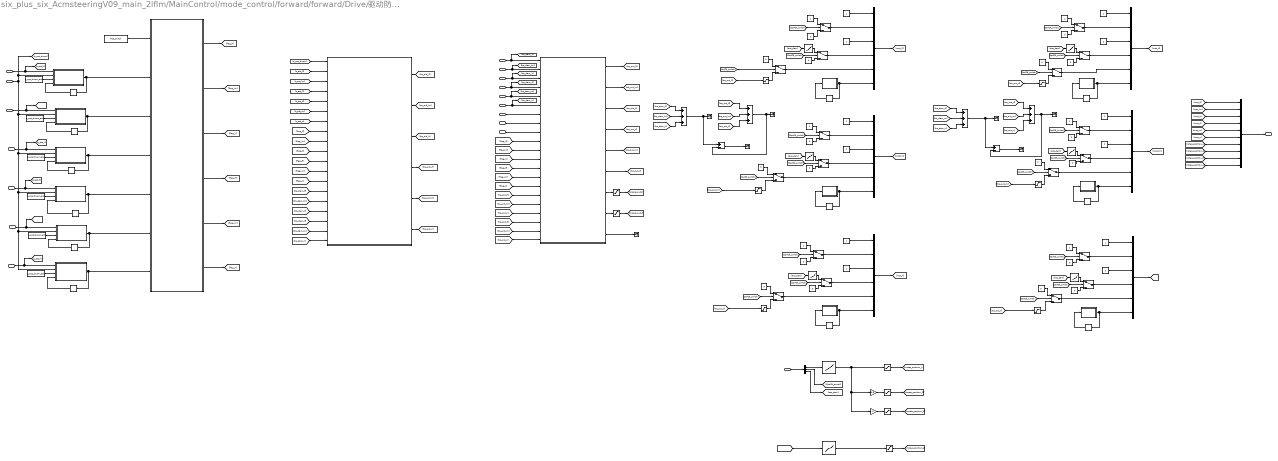
== system six_plus_six_AcmsteeringV09_main_2lflm/MainControl/mode_control/forward/forward/Drive/驱动防滑控制TCS/直行TCS/直行 ==
  trq_dem_lf : Inport
  trq_dem_lm : Inport  Port=2
  trq_dem_lr : Inport  Port=3
  trq_dem_rf : Inport  Port=4
  trq_dem_rm : Inport  Port=5
  trq_dem_rr : Inport  Port=6
  bra_pre_l : Inport  Port=7
  bra_pre_r : Inport  Port=8
  s_act_lf : Inport  Port=9
  s_act_lm : Inport  Port=10
  s_act_lr : Inport  Port=11
  s_act_rf : Inport  Port=12
  s_act_rm : Inport  Port=13
  s_act_rr : Inport  Port=14
  brake_dem : Inport  Port=15
  s_opt_zhuan : Inport  Port=16
  Signals : Inport  Port=17
  1-D Lookup Table : Lookup_n-D  NumberOfTableDimensions=1  BreakpointsForDimension1=zhuanxiang_youmen  Table=zhuanxiang_bianmazhi  InternalRulePriority=Speed  RndMeth=Simplest  InputSameDT=on
  1-D Lookup Table1 : Lookup_n-D  NumberOfTableDimensions=1  BreakpointsForDimension1=zhidong_youmen  Table=zhidong_bianmazhi  InternalRulePriority=Speed  RndMeth=Simplest  InputSameDT=on
  1-D Lookup Table{2..7} (6 alike) : Lookup_n-D  NumberOfTableDimensions=1  BreakpointsForDimension1=acc_spdctl  Table=spd_spdctl  InternalRulePriority=Speed  RndMeth=Simplest  InputSameDT=on
  Add{,1..3} (4 alike) : Sum  Inputs=+++
  Bus Selector : BusSelector  OutputSignals=RemoteControl_dem.steer_dem,RemoteControl_dem.SpdCtl_switch,RemoteControl_dem.acc_dem
  Constant{,1,3..6} (6 alike) : Constant  Value=0  OutDataTypeStr=single  SampleTime=-1
  Constant{7..10,12..13} (6 alike) : Constant  Value=s_opt_zhuan_add  OutDataTypeStr=single  SampleTime=-1
  Constant11 : Constant  Value=TCS_switch  OutDataTypeStr=single  SampleTime=-1
  Gain : Gain  Gain=0.5
  Gain1 : Gain  Gain=-1
  HeartBeat : MATLAB Function  TreatAsAtomicUnit=on
  HeartBeat1 : MATLAB Function  TreatAsAtomicUnit=on
  HeartBeat2 : MATLAB Function  TreatAsAtomicUnit=on
  HeartBeat3 : MATLAB Function  TreatAsAtomicUnit=on
  HeartBeat4 : MATLAB Function  TreatAsAtomicUnit=on
  HeartBeat5 : MATLAB Function  TreatAsAtomicUnit=on
  MATLAB Function : MATLAB Function  TreatAsAtomicUnit=on
  MATLAB Function1 : MATLAB Function  TreatAsAtomicUnit=on
  MATLAB Function2 : MATLAB Function  TreatAsAtomicUnit=on
  MATLAB Function3 : MATLAB Function  TreatAsAtomicUnit=on
  MATLAB Function4 : MATLAB Function  TreatAsAtomicUnit=on
  MATLAB Function5 : MATLAB Function  TreatAsAtomicUnit=on
  MATLAB Function6 : MATLAB Function  TreatAsAtomicUnit=on
  MATLAB Function7 : MATLAB Function  TreatAsAtomicUnit=on
  Memory{,1..11} (12 alike) : Memory  InheritSampleTime=on
  Mux : Mux  Inputs=10
  Mux{1..6} (6 alike) : Mux  Inputs=6
  Saturation{,1..3,6..7} (6 alike) : Saturate  UpperLimit=trqmax_zx  LowerLimit=trqmaxneg  OutDataTypeStr=single
  Saturation10 : Saturate  UpperLimit=zhuanxiang_up  LowerLimit=zhuanxiang_down
  Saturation11 : Saturate  UpperLimit=zhidong_up  LowerLimit=zhidong_down
  Saturation4 : Saturate  UpperLimit=premax  LowerLimit=0
  Saturation5 : Saturate  UpperLimit=premax  LowerLimit=0
  Saturation8 : Saturate  UpperLimit=zhuanxiang_up  LowerLimit=zhuanxiang_down
  Saturation9 : Saturate  UpperLimit=zhuanxiang_up  LowerLimit=zhuanxiang_down
  SpdSet_dem{,1..5} (6 alike) : Constant  Value=0  OutDataTypeStr=single  SampleTime=-1
  Subsystem : Subsystem
  Subtract : Sum  Inputs=+-
  Subtract1 : Sum  Inputs=+-
  Switch{,1..17} (18 alike) : Switch  Criteria=u2 > Threshold  Threshold=0.5
  Terminator{1..7} (7 alike) : Terminator
  mot_enable{1..6} (6 alike) : Constant  OutDataTypeStr=single  SampleTime=-1
  mot_gear : Constant  OutDataTypeStr=single  SampleTime=-1
  mot_gear1 : Constant  Value=2  OutDataTypeStr=single  SampleTime=-1
  mot_gear2 : Constant  OutDataTypeStr=single  SampleTime=-1
  mot_gear3 : Constant  Value=2  OutDataTypeStr=single  SampleTime=-1
  mot_gear4 : Constant  OutDataTypeStr=single  SampleTime=-1
  mot_gear5 : Constant  Value=2  OutDataTypeStr=single  SampleTime=-1
  mot_mode{,1..5} (6 alike) : Constant  Value=0  OutDataTypeStr=single  SampleTime=-1
  mot_mode{6..11} (6 alike) : Constant  OutDataTypeStr=single  SampleTime=-1
  forward_dem : Outport
  wires:
  Mux/1 -> forward_dem/1
  Memory4/1 -> HeartBeat/1(life_pre)
  HeartBeat/1(life) -> Memory4/1, Mux1/6
  Mux1/1 -> [mot_lf]
  [trq_out_lf] -> Saturation/1  "trq_out_lf_forward"
  mot_gear/1 -> Mux1/3
  mot_enable4/1 -> Mux1/1
  Switch1/1 -> Mux1/4
  Memory1/1 -> HeartBeat2/1(life_pre)
  HeartBeat2/1(life) -> Mux3/6, Memory1/1
  Mux3/1 -> [mot_rf]
  [trq_out_rf] -> Saturation2/1  "trq_out_rf_forward"
  Switch3/1 -> Mux3/2
  mot_gear1/1 -> Mux3/3
  mot_enable2/1 -> Mux3/1
  Switch8/1 -> Mux3/4
  Memory2/1 -> HeartBeat3/1(life_pre)
  HeartBeat3/1(life) -> Mux5/6, Memory2/1
  Mux5/1 -> [mot_lm]
  [trq_out_lm] -> Saturation6/1  "trq_out_lm_forward"
  Switch4/1 -> Mux5/2
  mot_gear2/1 -> Mux5/3
  mot_enable5/1 -> Mux5/1
  Switch10/1 -> Mux5/4
  Memory3/1 -> HeartBeat4/1(life_pre)
  HeartBeat4/1(life) -> Memory3/1, Mux6/6
  Mux6/1 -> [mot_rm]
  [trq_out_rm] -> Saturation7/1  "trq_out_rm_forward"
  Switch5/1 -> Mux6/2
  mot_gear3/1 -> Mux6/3
  mot_enable6/1 -> Mux6/1
  Switch11/1 -> Mux6/4
  Memory5/1 -> HeartBeat1/1(life_pre)
  HeartBeat1/1(life) -> Mux2/6, Memory5/1
  Mux2/1 -> [mot_lr]
  [trq_out_lr] -> Saturation1/1  "trq_out_lr_forward"
  Switch6/1 -> Mux2/2
  mot_gear4/1 -> Mux2/3
  mot_enable1/1 -> Mux2/1
  Switch12/1 -> Mux2/4
  Memory6/1 -> HeartBeat5/1(life_pre)
  HeartBeat5/1(life) -> Memory6/1, Mux4/6
  Mux4/1 -> [mot_rr]
  [trq_out_rr] -> Saturation3/1  "trq_out_rr_forward"
  Switch7/1 -> Mux4/2
  mot_gear5/1 -> Mux4/3
  mot_enable3/1 -> Mux4/1
  Switch13/1 -> Mux4/4
  [mot_lf] -> Mux/1
  [mot_lm] -> Mux/2
  [mot_lr] -> Mux/3
  [mot_rf] -> Mux/4
  [mot_rm] -> Mux/5
  [mot_rr] -> Mux/6
  [motec_position_1] -> Mux/7
  [motec_position_2] -> Mux/8
  [motec_position_3] -> Mux/9
  1-D Lookup Table1/1 -> Saturation11/1
  1-D Lookup Table/1 -> Gain1/1, Gain/1, Saturation8/1
  Signals/1 -> Bus Selector/1
  Gain1/1 -> Saturation10/1
  Bus Selector/1 -> 1-D Lookup Table/1  "<steer_dem>"
  Gain/1 -> Saturation9/1
  Saturation8/1 -> [motec_position_1]
  Saturation9/1 -> [motec_position_2]
  Saturation10/1 -> [motec_position_3]
  Saturation11/1 -> [motec_position_4]
  [brapre_out_l] -> 1-D Lookup Table1/1
  [motec_position_4] -> Mux/10
  Bus Selector/2 -> [SpdCtl_switch]  "<SpdCtl_switch>"
  [SpdCtl_switch] -> Switch/2
  mot_mode6/1 -> Switch/1
  mot_mode/1 -> Switch/3
  Switch/1 -> Mux1/2
  [SpdCtl_switch] -> Switch1/2
  SpdSet_dem/1 -> Switch1/3
  Bus Selector/3 -> [acc_dem]  "<acc_dem>"
  [acc_dem] -> 1-D Lookup Table2/1
  1-D Lookup Table2/1 -> Switch1/1
  [SpdCtl_switch] -> Switch2/2
  Saturation/1 -> Switch2/3
  Constant/1 -> Switch2/1
  Switch2/1 -> Mux1/5
  [SpdCtl_switch] -> Switch3/2
  mot_mode7/1 -> Switch3/1
  mot_mode2/1 -> Switch3/3
  [SpdCtl_switch] -> Switch4/2
  mot_mode8/1 -> Switch4/1
  mot_mode4/1 -> Switch4/3
  [SpdCtl_switch] -> Switch5/2
  mot_mode9/1 -> Switch5/1
  mot_mode5/1 -> Switch5/3
  [SpdCtl_switch] -> Switch6/2
  mot_mode10/1 -> Switch6/1
  mot_mode1/1 -> Switch6/3
  [SpdCtl_switch] -> Switch7/2
  mot_mode11/1 -> Switch7/1
  mot_mode3/1 -> Switch7/3
  [SpdCtl_switch] -> Switch8/2
  [acc_dem] -> 1-D Lookup Table3/1
  1-D Lookup Table3/1 -> Switch8/1
  SpdSet_dem1/1 -> Switch8/3
  [SpdCtl_switch] -> Switch9/2
  Constant1/1 -> Switch9/1
  Saturation2/1 -> Switch9/3
  Switch9/1 -> Mux3/5
  [SpdCtl_switch] -> Switch10/2
  [acc_dem] -> 1-D Lookup Table4/1
  1-D Lookup Table4/1 -> Switch10/1
  SpdSet_dem4/1 -> Switch10/3
  [SpdCtl_switch] -> Switch11/2
  [acc_dem] -> 1-D Lookup Table5/1
  1-D Lookup Table5/1 -> Switch11/1
  SpdSet_dem5/1 -> Switch11/3
  [SpdCtl_switch] -> Switch12/2
  [acc_dem] -> 1-D Lookup Table6/1
  1-D Lookup Table6/1 -> Switch12/1
  SpdSet_dem2/1 -> Switch12/3
  [SpdCtl_switch] -> Switch13/2
  [acc_dem] -> 1-D Lookup Table7/1
  1-D Lookup Table7/1 -> Switch13/1
  SpdSet_dem3/1 -> Switch13/3
  [SpdCtl_switch] -> Switch14/2
  Constant3/1 -> Switch14/1
  Saturation6/1 -> Switch14/3
  Switch14/1 -> Mux5/5
  [SpdCtl_switch] -> Switch15/2
  Constant4/1 -> Switch15/1
  Saturation7/1 -> Switch15/3
  Switch15/1 -> Mux6/5
  [SpdCtl_switch] -> Switch16/2
  Constant5/1 -> Switch16/1
  Saturation1/1 -> Switch16/3
  Switch16/1 -> Mux2/5
  [SpdCtl_switch] -> Switch17/2
  Constant6/1 -> Switch17/1
  Saturation3/1 -> Switch17/3
  Switch17/1 -> Mux4/5
  Constant10/1 -> MATLAB Function3/3(s_opt_zhuan_add)
  Memory9/1 -> MATLAB Function3/4(flag_rr_pre)
  MATLAB Function3/1(flag_rr) -> Memory9/1, MATLAB Function5/7(flag_rr)
  s_act_rr/1 -> [s_act_rr], MATLAB Function3/1(s_act_rr)
  Constant9/1 -> MATLAB Function2/3(s_opt_zhuan_add)
  Memory8/1 -> MATLAB Function2/4(flag_rf_pre)
  MATLAB Function2/1(flag_rf) -> Memory8/1, MATLAB Function5/5(flag_rf)
  s_act_rf/1 -> MATLAB Function2/1(s_act_rf), [s_act_rf]
  Constant8/1 -> MATLAB Function1/3(s_opt_zhuan_add)
  Memory7/1 -> MATLAB Function1/4(flag_lr_pre)
  MATLAB Function1/1(flag_lr) -> Memory7/1, MATLAB Function5/4(flag_lr)
  s_act_lr/1 -> [s_act_lr], MATLAB Function1/1(s_act_lr)
  Constant7/1 -> MATLAB Function/3(s_opt_zhuan_add)
  Memory/1 -> MATLAB Function/4(flag_lf_pre)
  MATLAB Function/1(flag_lf) -> Memory/1, MATLAB Function5/2(flag_lf)
  s_act_lf/1 -> [s_act_lf], MATLAB Function/1(s_act_lf)
  [trq_dem_lf] -> Subsystem/14(trq_dem_lf)
  [flag_lf] -> Subsystem/8(flag_lf)
  [trq_dem_rf] -> Subsystem/17(trq_dem_rf)
  [trq_dem_lr] -> Subsystem/16(trq_dem_lr)
  [flag_lr] -> Subsystem/10(flag_lr)
  [flag_rf] -> Subsystem/11(flag_rf)
  [trq_dem_rr] -> Subsystem/19(trq_dem_rr)
  [flag_rr] -> Subsystem/13(flag_rr)
  [s_opt_zhuan] -> Subsystem/1(s_opt_zhuan)
  [s_act_rr] -> Subsystem/7(s_act_rr)
  [s_act_rf] -> Subsystem/5(s_act_rf)
  [s_act_lr] -> Subsystem/4(s_act_lr)
  [s_act_lf] -> Subsystem/2(s_act_lf)
  Subsystem/3(trq_pid_lr) -> [trq_pid_lr]
  Subsystem/1(trq_pid_lf) -> [trq_pid_lf]
  Subsystem/6(trq_pid_rr) -> [trq_pid_rr]
  Subsystem/4(trq_pid_rf) -> [trq_pid_rf]
  MATLAB Function5/1(flag_lf1) -> [flag_lf]  "flag_lf"
  MATLAB Function5/3(flag_lr1) -> [flag_lr]  "flag_lr"
  MATLAB Function5/4(flag_rf1) -> [flag_rf]  "flag_rf"
  MATLAB Function5/6(flag_rr1) -> [flag_rr]  "flag_rr"
  Constant12/1 -> MATLAB Function4/3(s_opt_zhuan_add)
  Memory10/1 -> MATLAB Function4/4(flag_lm_pre)
  MATLAB Function4/1(flag_lm) -> MATLAB Function5/3(flag_lm), Memory10/1
  s_act_lm/1 -> MATLAB Function4/1(s_act_lm), [s_act_lm]
  Constant13/1 -> MATLAB Function6/3(s_opt_zhuan_add)
  Memory11/1 -> MATLAB Function6/4(flag_rm_pre)
  MATLAB Function6/1(flag_rm) -> Memory11/1, MATLAB Function5/6(flag_rm)
  s_act_rm/1 -> [s_act_rm], MATLAB Function6/1(s_act_rm)
  s_opt_zhuan/1 -> MATLAB Function/2(s_opt_zhuan), [s_opt_zhuan], MATLAB Function4/2(s_opt_zhuan), MATLAB Function1/2(s_opt_zhuan), MATLAB Function2/2(s_opt_zhuan), MATLAB Function6/2(s_opt_zhuan), MATLAB Function3/2(s_opt_zhuan)
  MATLAB Function5/2(flag_lm1) -> [flag_lm]  "flag_lm"
  MATLAB Function5/5(flag_rm1) -> [flag_rm]  "flag_rm"
  Constant11/1 -> MATLAB Function5/1(TCS_switch)
  [s_act_lm] -> Subsystem/3(s_act_lm)
  [s_act_rm] -> Subsystem/6(s_act_rm)
  [flag_lm] -> Subsystem/9(flag_lm)
  [flag_rm] -> Subsystem/12(flag_rm)
  [trq_dem_lm] -> Subsystem/15(trq_dem_lm)
  [trq_dem_rm] -> Subsystem/18(trq_dem_rm)
  Subsystem/2(trq_pid_lm) -> [trq_pid_lm]
  Subsystem/5(trq_pid_rm) -> [trq_pid_rm]
  [flag_rr] -> MATLAB Function7/15(flag_rr)
  [flag_rf] -> MATLAB Function7/13(flag_rf)
  [flag_lr] -> MATLAB Function7/12(flag_lr)
  [flag_lf] -> MATLAB Function7/10(flag_lf)
  [trq_pid_lf] -> MATLAB Function7/16(trq_pid_lf)
  [trq_pid_lr] -> MATLAB Function7/18(trq_pid_lr)
  [trq_pid_rf] -> MATLAB Function7/19(trq_pid_rf)
  [trq_pid_rr] -> MATLAB Function7/21(trq_pid_rr)
  trq_dem_lf/1 -> MATLAB Function7/1(trq_dem_lf), [trq_dem_lf]
  trq_dem_lr/1 -> [trq_dem_lr], MATLAB Function7/3(trq_dem_lr)
  trq_dem_rf/1 -> MATLAB Function7/4(trq_dem_rf), [trq_dem_rf]
  trq_dem_rr/1 -> [trq_dem_rr], MATLAB Function7/6(trq_dem_rr)
  bra_pre_l/1 -> MATLAB Function7/7(bra_pre_l)
  bra_pre_r/1 -> MATLAB Function7/8(bra_pre_r)
  MATLAB Function7/1(trq_out_lf) -> [trq_out_lf]
  MATLAB Function7/3(trq_out_lr) -> [trq_out_lr]
  MATLAB Function7/4(trq_out_rf) -> [trq_out_rf]
  MATLAB Function7/6(trq_out_rr) -> [trq_out_rr]
  MATLAB Function7/7(brapre_out_l) -> Saturation4/1
  MATLAB Function7/8(brapre_out_r) -> Saturation5/1
  brake_dem/1 -> MATLAB Function7/9(brake_dem)
  MATLAB Function7/9(mode) -> Terminator2/1  "TCS_mode"
  Saturation4/1 -> [brapre_out_l]
  Saturation5/1 -> [brapre_out_r]
  MATLAB Function7/2(trq_out_lm) -> [trq_out_lm]
  MATLAB Function7/5(trq_out_rm) -> [trq_out_rm]
  trq_dem_lm/1 -> [trq_dem_lm], MATLAB Function7/2(trq_dem_lm)
  trq_dem_rm/1 -> [trq_dem_rm], MATLAB Function7/5(trq_dem_rm)
  [flag_lm] -> MATLAB Function7/11(flag_lm)
  [flag_rm] -> MATLAB Function7/14(flag_rm)
  [trq_pid_lm] -> MATLAB Function7/17(trq_pid_lm)
  [trq_pid_rm] -> MATLAB Function7/20(trq_pid_rm)
  [trq_out_lm] -> Add/2
  [trq_out_lf] -> Add/1
  [trq_out_lr] -> Add/3
  Add/1 -> Subtract/2, Terminator1/1  "trq_out_l_forward"
  [trq_out_rm] -> Add1/2
  [trq_out_rf] -> Add1/1
  [trq_out_rr] -> Add1/3
  Add1/1 -> Subtract1/2, Terminator3/1  "trq_out_r_forward"
  [trq_dem_lm] -> Add2/2
  [trq_dem_lr] -> Add2/3
  [trq_dem_lf] -> Add2/1
  Add2/1 -> Subtract/1, Terminator4/1  "trq_dem_l_forward"
  Subtract/1 -> Terminator5/1  "trq_adjust_l_forward"
  [trq_dem_rm] -> Add3/2
  [trq_dem_rf] -> Add3/1
  [trq_dem_rr] -> Add3/3
  Add3/1 -> Subtract1/1, Terminator6/1  "trq_dem_r_forward"
  Subtract1/1 -> Terminator7/1  "trq_adjust_r_forward"

== system six_plus_six_AcmsteeringV09_main_2lflm/MainControl/mode_control/backward/backward/Drive/驱动防滑控制TCS/直行TCS/直行/Subsystem ==
  s_opt_zhuan : Inport
  s_act_lf : Inport  Port=2
  s_act_lm : Inport  Port=3
  s_act_lr : Inport  Port=4
  s_act_rf : Inport  Port=5
  s_act_rm : Inport  Port=6
  s_act_rr : Inport  Port=7
  flag_lf : Inport  Port=8
  flag_lm : Inport  Port=9
  flag_lr : Inport  Port=10
  flag_rf : Inport  Port=11
  flag_rm : Inport  Port=12
  flag_rr : Inport  Port=13
  trq_dem_lf : Inport  Port=14
  trq_dem_lm : Inport  Port=15
  trq_dem_lr : Inport  Port=16
  trq_dem_rf : Inport  Port=17
  trq_dem_rm : Inport  Port=18
  trq_dem_rr : Inport  Port=19
  If{,1..5} (6 alike) : If  IfExpression=u1 > 0.5  ShowElse=off
  Subsystem : Subsystem
  Subsystem1 : Subsystem
  Subsystem2 : Subsystem
  Subsystem3 : Subsystem
  Subsystem4 : Subsystem
  Subsystem5 : Subsystem
  Switch{,1..5} (6 alike) : Switch  Criteria=u2 > Threshold  Threshold=0.5  OutDataTypeStr=single
  trq_pid_lf : Outport
  trq_pid_lm : Outport  Port=2
  trq_pid_lr : Outport  Port=3
  trq_pid_rf : Outport  Port=4
  trq_pid_rm : Outport  Port=5
  trq_pid_rr : Outport  Port=6
  wires:
  Switch/1 -> trq_pid_lf/1
  trq_dem_rr/1 -> Switch2/3, Subsystem3/3(trq_dem_rr)
  flag_rr/1 -> [flag_rr], Switch2/2
  Switch2/1 -> trq_pid_rr/1
  trq_dem_rf/1 -> Subsystem2/3(trq_dem_rf), Switch3/3
  flag_rf/1 -> [flag_rf], Switch3/2
  Switch3/1 -> trq_pid_rf/1
  s_act_lf/1 -> Subsystem/2(s_act_lf)
  Subsystem/1(trq_pid_lf) -> Switch/1
  If/1 -> Subsystem/Action
  flag_lf/1 -> [flag_lf], Switch/2
  trq_dem_lf/1 -> Switch/3, Subsystem/3(trq_dem_lf)
  Switch1/1 -> trq_pid_lr/1
  s_opt_zhuan/1 -> [s_opt_zhuan], Subsystem/1(s_opt_zhuan)
  s_act_lr/1 -> Subsystem1/2(s_act_lr)
  Subsystem1/1(trq_pid_lr) -> Switch1/1
  If1/1 -> Subsystem1/Action
  flag_lr/1 -> [flag_lr], Switch1/2
  trq_dem_lr/1 -> Switch1/3, Subsystem1/3(trq_dem_lr)
  s_act_rf/1 -> Subsystem2/2(s_act_rf)
  Subsystem2/1(trq_pid_rf) -> Switch3/1
  If2/1 -> Subsystem2/Action
  s_act_rr/1 -> Subsystem3/2(s_act_rr)
  Subsystem3/1(trq_pid_rr) -> Switch2/1
  If3/1 -> Subsystem3/Action
  [flag_lf] -> If/1
  [s_opt_zhuan] -> Subsystem2/1(s_opt_zhuan)
  [s_opt_zhuan] -> Subsystem1/1(s_opt_zhuan)
  [s_opt_zhuan] -> Subsystem3/1(s_opt_zhuan)
  [flag_lr] -> If1/1
  [flag_rf] -> If2/1
  Switch4/1 -> trq_pid_lm/1
  s_act_lm/1 -> Subsystem4/2(s_act_lm)
  Subsystem4/1(trq_pid_lm) -> Switch4/1
  If4/1 -> Subsystem4/Action
  flag_lm/1 -> Switch4/2, [flag_lm]
  trq_dem_lm/1 -> Subsystem4/3(trq_dem_lm), Switch4/3
  [s_opt_zhuan] -> Subsystem4/1(s_opt_zhuan)
  [flag_lm] -> If4/1
  trq_dem_rm/1 -> Switch5/3, Subsystem5/3(trq_dem_rm)
  flag_rm/1 -> Switch5/2, [flag_rm]
  Switch5/1 -> trq_pid_rm/1
  s_act_rm/1 -> Subsystem5/2(s_act_rm)
  Subsystem5/1(trq_pid_rm) -> Switch5/1
  If5/1 -> Subsystem5/Action
  [s_opt_zhuan] -> Subsystem5/1(s_opt_zhuan)
  [flag_rm] -> If5/1
  [flag_rr] -> If3/1

== system six_plus_six_AcmsteeringV09_main_2lflm/MainControl/mode_control/forward/forward/Drive/驱动防滑控制TCS/直行TCS/直行/Subsystem ==
  s_opt_zhuan : Inport
  s_act_lf : Inport  Port=2
  s_act_lm : Inport  Port=3
  s_act_lr : Inport  Port=4
  s_act_rf : Inport  Port=5
  s_act_rm : Inport  Port=6
  s_act_rr : Inport  Port=7
  flag_lf : Inport  Port=8
  flag_lm : Inport  Port=9
  flag_lr : Inport  Port=10
  flag_rf : Inport  Port=11
  flag_rm : Inport  Port=12
  flag_rr : Inport  Port=13
  trq_dem_lf : Inport  Port=14
  trq_dem_lm : Inport  Port=15
  trq_dem_lr : Inport  Port=16
  trq_dem_rf : Inport  Port=17
  trq_dem_rm : Inport  Port=18
  trq_dem_rr : Inport  Port=19
  If{,1..5} (6 alike) : If  IfExpression=u1 > 0.5  ShowElse=off
  Subsystem : Subsystem
  Subsystem1 : Subsystem
  Subsystem2 : Subsystem
  Subsystem3 : Subsystem
  Subsystem4 : Subsystem
  Subsystem5 : Subsystem
  Switch{,1..5} (6 alike) : Switch  Criteria=u2 > Threshold  Threshold=0.5  OutDataTypeStr=single
  trq_pid_lf : Outport
  trq_pid_lm : Outport  Port=2
  trq_pid_lr : Outport  Port=3
  trq_pid_rf : Outport  Port=4
  trq_pid_rm : Outport  Port=5
  trq_pid_rr : Outport  Port=6
  wires:
  Switch/1 -> trq_pid_lf/1
  trq_dem_rr/1 -> Switch2/3, Subsystem3/3(trq_dem_rr)
  flag_rr/1 -> [flag_rr], Switch2/2
  Switch2/1 -> trq_pid_rr/1
  trq_dem_rf/1 -> Subsystem2/3(trq_dem_rf), Switch3/3
  flag_rf/1 -> [flag_rf], Switch3/2
  Switch3/1 -> trq_pid_rf/1
  s_act_lf/1 -> Subsystem/2(s_act_lf)
  Subsystem/1(trq_pid_lf) -> Switch/1
  If/1 -> Subsystem/Action
  flag_lf/1 -> [flag_lf], Switch/2
  trq_dem_lf/1 -> Switch/3, Subsystem/3(trq_dem_lf)
  Switch1/1 -> trq_pid_lr/1
  s_opt_zhuan/1 -> [s_opt_zhuan], Subsystem/1(s_opt_zhuan)
  s_act_lr/1 -> Subsystem1/2(s_act_lr)
  Subsystem1/1(trq_pid_lr) -> Switch1/1
  If1/1 -> Subsystem1/Action
  flag_lr/1 -> [flag_lr], Switch1/2
  trq_dem_lr/1 -> Switch1/3, Subsystem1/3(trq_dem_lr)
  s_act_rf/1 -> Subsystem2/2(s_act_rf)
  Subsystem2/1(trq_pid_rf) -> Switch3/1
  If2/1 -> Subsystem2/Action
  s_act_rr/1 -> Subsystem3/2(s_act_rr)
  Subsystem3/1(trq_pid_rr) -> Switch2/1
  If3/1 -> Subsystem3/Action
  [flag_lf] -> If/1
  [s_opt_zhuan] -> Subsystem2/1(s_opt_zhuan)
  [s_opt_zhuan] -> Subsystem1/1(s_opt_zhuan)
  [s_opt_zhuan] -> Subsystem3/1(s_opt_zhuan)
  [flag_lr] -> If1/1
  [flag_rf] -> If2/1
  Switch4/1 -> trq_pid_lm/1
  s_act_lm/1 -> Subsystem4/2(s_act_lm)
  Subsystem4/1(trq_pid_lm) -> Switch4/1
  If4/1 -> Subsystem4/Action
  flag_lm/1 -> Switch4/2, [flag_lm]
  trq_dem_lm/1 -> Subsystem4/3(trq_dem_lm), Switch4/3
  [s_opt_zhuan] -> Subsystem4/1(s_opt_zhuan)
  [flag_lm] -> If4/1
  trq_dem_rm/1 -> Switch5/3, Subsystem5/3(trq_dem_rm)
  flag_rm/1 -> Switch5/2, [flag_rm]
  Switch5/1 -> trq_pid_rm/1
  s_act_rm/1 -> Subsystem5/2(s_act_rm)
  Subsystem5/1(trq_pid_rm) -> Switch5/1
  If5/1 -> Subsystem5/Action
  [s_opt_zhuan] -> Subsystem5/1(s_opt_zhuan)
  [flag_rm] -> If5/1
  [flag_rr] -> If3/1
